simulink model "BZERO_MODEL"  (R2025b)
settings: Solver=ode23t  StartTime=0.0  StopTime=10000  RelTol=1e-3
InitFcn:
  | setup_bzero;
values from neighbouring files (symbols this model uses):
  bike_mass = 220    [setup_bzero.m]
  finish_line = track_dist(end)    [setup_bzero.m]
  g = 9.81    [Fly_lap.m]    (also in setup_bzero.m)
  L = 2    [setup_bzero.m]
  Max_brake_pressure_F_Bar = 70    [setup_bzero.m]
  Max_brake_pressure_R_Bar = 20    [setup_bzero.m]
  mot_rpm_vec = [0, 250, 500, 750, 1000, 1250, 1500, 1750, 2000, 2250, 2500, 2750, 3000, 3250, 3500, 3750, 4000, 4250, 4500, 4750, 5000, 5250, 5500, 5750, 6000, 6250, 6500, 6750, 7000, 7250, 7500]    [setup_bzero.m]
  mot_trq_vec = [120, 120, 120, 120, 120, 120, 120, 120, 120, 120, 120, 120, 120, 120, 120, 120, 114.592, 107.851, 101.859, 96.498, 91.673, 87.308, 83.339, 79.716, 76.394, 73.339, 70.518, 67.906, 65.481, 63.223, 61.115]    [setup_bzero.m]
  Np = 12    [setup_bzero.m]
  Ns = 28    [setup_bzero.m]
  regen_bias = 0.2    [setup_bzero.m]
  s = surf(X_surf, Y_surf, Z_surf, Z_surf)    [Fly_lap.m]
  target_vel = data.Velocity_ms    [setup_bzero.m]
  track_dist = data.Distance_m    [setup_bzero.m]
  track_grade = data.Grade_rad    [setup_bzero.m]
  V_init = 117    [setup_bzero.m]
  v_init = target_vel(1)    [setup_bzero.m]
undefined symbols (not defined in the file or in its folder): Driver_Ki, Driver_Kp, Neg, Pos
libraries: fl_lib x20, nesl_utility x13, sdl_lib x7, batteryecm_lib x1, autolibshared x1
(part 2 of 2)

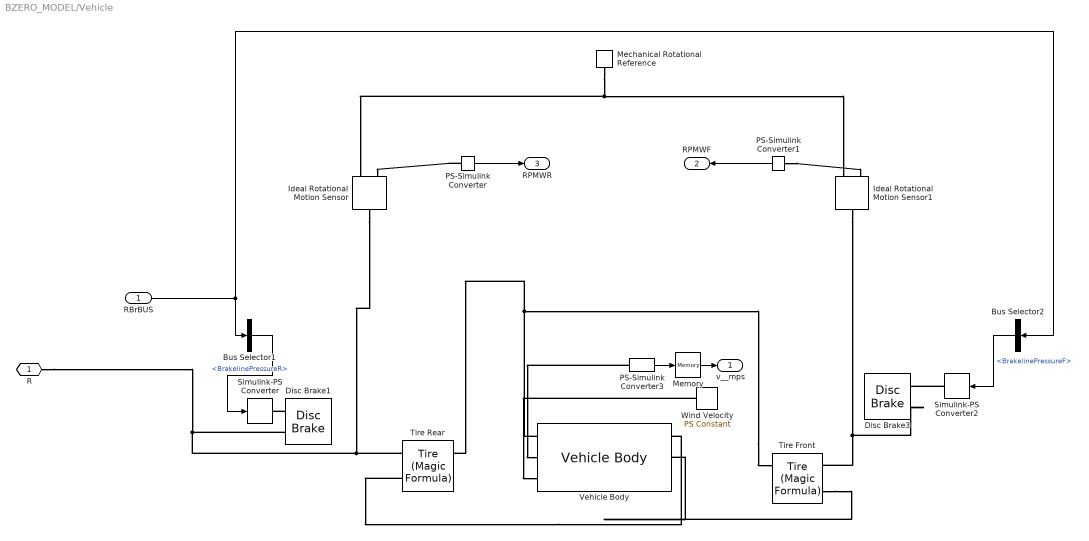
== system BZERO_MODEL/Vehicle ==
  RBrBUS : Inport
  Bus Selector1 : BusSelector  OutputSignals=BrakelinePressureR
  Bus Selector2 : BusSelector  OutputSignals=BrakelinePressureF
  Disc Brake1 : sdl_lib/Brakes & Detents/Rotational/Disc Brake  r_mean=R_eff m  bore=D_piston m  n_pads=2  thermal_port=simscape.enum.thermaleffects.omit  mu_static=Static_Cf  mu_coulomb=mu_pad  temperature_TLU=[280, 300, 320] K  mu_static_TLU=[.9, .8, .7]  mu_coulomb_TLU=[.8, .7, .6]  brkwy_vel=Break_Fric_v_rads rad/s  visc_coef=Viscous_Cf N*m*s/rad  thermal_mass=50 kJ/K  temperature_specify=off  temperature_priority=High  temperature=300 K  temperature_nominal_specify=off  temperature_nominal_value=1  temperature_nominal_unit=K
  Disc Brake3 : sdl_lib/Brakes & Detents/Rotational/Disc Brake  r_mean=R_eff m  bore=D_piston m  n_pads=2  thermal_port=simscape.enum.thermaleffects.omit  mu_static=Static_Cf  mu_coulomb=mu_pad  temperature_TLU=[280, 300, 320] K  mu_static_TLU=[.9, .8, .7]  mu_coulomb_TLU=[.8, .7, .6]  brkwy_vel=Break_Fric_v_rads rad/s  visc_coef=Viscous_Cf N*m*s/rad  thermal_mass=50 kJ/K  temperature_specify=off  temperature_priority=High  temperature=300 K  temperature_nominal_specify=off  temperature_nominal_value=1  temperature_nominal_unit=K
  Ideal Rotational Motion Sensor : fl_lib/Mechanical/Mechanical Sensors/Ideal Rotational Motion Sensor  reference=foundation.enum.MeasurementReference.difference  acceleration_port=false  velocity_port=true  position_port=false  wrap_angle=false  offset=0 rad
      settings: InternalSimscapePortConfiguration="{\"Bottom\":[],\"Left\":[{\"id\":\"R\",\"label\":\"R\",\"type\":\"foundation.mechanical.rotational.rotational\"}],\"Right\":[{\"id\":\"C\",\"label\":\"C\",\"type\":\"foundation.mechanical.rotational.rotational\"},{\"id\":\"W\",\"label\":\"W\",\"type\":\"output\"}],\"Top\":[]}"
  Ideal Rotational Motion Sensor1 : fl_lib/Mechanical/Mechanical Sensors/Ideal Rotational Motion Sensor  reference=foundation.enum.MeasurementReference.difference  acceleration_port=false  velocity_port=true  position_port=false  wrap_angle=false  offset=0 rad
      settings: InternalSimscapePortConfiguration="{\"Bottom\":[],\"Left\":[{\"id\":\"R\",\"label\":\"R\",\"type\":\"foundation.mechanical.rotational.rotational\"}],\"Right\":[{\"id\":\"C\",\"label\":\"C\",\"type\":\"foundation.mechanical.rotational.rotational\"},{\"id\":\"W\",\"label\":\"W\",\"type\":\"output\"}],\"Top\":[]}"
  Mechanical Rotational Reference : fl_lib/Mechanical/Rotational Elements/Mechanical Rotational Reference
  Memory : Memory  InitialCondition=v_init  LinearizeMemory=on  LinearizeAsDelay=on
  PS-Simulink Converter : nesl_utility/PS-Simulink Converter  PhysicalDomain=network_engine_domain  SubClassName=ps_output  LeftPortType=input  RightPortType=output  PseudoPeriodic=off  Frequencies=[]  VectorFormat=inherit  Unit=rpm  AffineConversion=off
  PS-Simulink Converter1 : nesl_utility/PS-Simulink Converter  PhysicalDomain=network_engine_domain  SubClassName=ps_output  LeftPortType=input  RightPortType=output  PseudoPeriodic=off  Frequencies=[]  VectorFormat=inherit  Unit=rpm  AffineConversion=off
  PS-Simulink Converter3 : nesl_utility/PS-Simulink Converter  PhysicalDomain=network_engine_domain  SubClassName=ps_output  LeftPortType=input  RightPortType=output  PseudoPeriodic=off  Frequencies=[]  VectorFormat=1-D array  Unit=m/s  AffineConversion=off
  Simulink-PS Converter : nesl_utility/Simulink-PS Converter  PhysicalDomain=network_engine_domain  SubClassName=ps_input  LeftPortType=input  RightPortType=output  PseudoPeriodic=off  Frequencies=[]  NoiseDistribution=none  NoiseParameters=[]  Unit=Pa  AffineConversion=off  FilteringAndDerivatives=zero  SimscapeFilterOrder=1  InputFilterTimeConstant=.001  UdotUserProvided=0
  Simulink-PS Converter2 : nesl_utility/Simulink-PS Converter  PhysicalDomain=network_engine_domain  SubClassName=ps_input  LeftPortType=input  RightPortType=output  PseudoPeriodic=off  Frequencies=[]  NoiseDistribution=none  NoiseParameters=[]  Unit=Pa  AffineConversion=off  FilteringAndDerivatives=zero  SimscapeFilterOrder=1  InputFilterTimeConstant=.001  UdotUserProvided=0
  Tire Front : sdl_lib/Tires & Vehicles/Tire (Magic Formula)  parameterization=sdl.enum.magic_tire_model.peak  F_z1=Fz_rated N  F_x1=Fx_peak N  kappa1=slip_peak  B_m=10  C_m=1.9  D_m=1  E_m=0.97  fz0=4e+3 N  p_Cx=1.685  p_Dx=[ 1.21 -0.037 ]  p_Ex=[ 0.344 0.095 -0.02 0 ]  p_Kx=[ 21.51 -0.163 0.245 ]  p_Hx=[ -0.002 0.002 ]  p_Vx=[ 0 0 ]  rolling_radius_model=sdl.enum.RollingRadiusParameterization.Constant  r_e=wheel_radius m  r_0=0.3 m  breff=8.39  dreff=0.26  freff=0.074  q_re0=0.99  q_v1=0.008  longvl=17 m/s  cz=5e5 N/m  model_resistance=true  resistance_model=1  coeff=Ad  p_tire=2.5e+5 Pa  alpha=-0.003  beta=0.97  coeff_a=0.008399999999999999  coeff_b=6.2e-4 s/m  coeff_c=1.6e-4 s^2/m^2  p_tire0=240e3 Pa  fz0_resistance=4000 N  vH0=16 m/s  q_Sy=[.0082, 0, .0014, .001, 0, 0, 1.08, -.5]  v_thr=0.001 m/s  enable_scaling_coefficients=false  lfzO=1  lcx=1  lmux=1  lex=1  lkx=1  lhx=1  lvx=1  lmy=1  model_compliance=sdl.enum.compliance.off  stiffness=1e+6 N/m  damping=1000 N/(m/s)  model_inertia=1  inertia=I_wheel_front kg*m^2  initial_velocity=wheel_rpm_init rpm  vxlow=0.1 m/s  v_tr_thr=0.1*(0.1) m/s  kpumin=-1e5  kpumax=1e8
  Tire Rear : sdl_lib/Tires & Vehicles/Tire (Magic Formula)  parameterization=sdl.enum.magic_tire_model.peak  F_z1=Fz_rated N  F_x1=Fx_peak N  kappa1=slip_peak  B_m=10  C_m=1.9  D_m=1  E_m=0.97  fz0=4e+3 N  p_Cx=1.685  p_Dx=[ 1.21 -0.037 ]  p_Ex=[ 0.344 0.095 -0.02 0 ]  p_Kx=[ 21.51 -0.163 0.245 ]  p_Hx=[ -0.002 0.002 ]  p_Vx=[ 0 0 ]  rolling_radius_model=sdl.enum.RollingRadiusParameterization.Constant  r_e=wheel_radius m  r_0=0.3 m  breff=8.39  dreff=0.26  freff=0.074  q_re0=0.99  q_v1=0.008  longvl=17 m/s  cz=5e5 N/m  model_resistance=true  resistance_model=sdl.enum.rollingResistanceParameterization.constant  coeff=Ad  p_tire=2.5e+5 Pa  alpha=-0.003  beta=0.97  coeff_a=0.008399999999999999  coeff_b=6.2e-4 s/m  coeff_c=1.6e-4 s^2/m^2  p_tire0=240e3 Pa  fz0_resistance=4000 N  vH0=16 m/s  q_Sy=[.0082, 0, .0014, .001, 0, 0, 1.08, -.5]  v_thr=0.001 m/s  enable_scaling_coefficients=false  lfzO=1  lcx=1  lmux=1  lex=1  lkx=1  lhx=1  lvx=1  lmy=1  model_compliance=sdl.enum.compliance.off  stiffness=1e+6 N/m  damping=1000 N/(m/s)  model_inertia=1  inertia=I_wheel_rear kg*m^2  initial_velocity=wheel_rpm_init rpm  vxlow=0.1 m/s  v_tr_thr=0.1*(0.1) m/s  kpumin=-1e5  kpumax=1e8
  Vehicle Body : sdl_lib/Tires & Vehicles/Vehicle Body  mass=bike_mass kg  n_w=1  x_f=D_CoG_F_m m  x_r=D_CoG_R_m m  y_c=H_CoG_m m  mass_var=simscape.enum.onoff.off  g=g m/s^2  liftoff_warning=0  area=frontal_area m^2  Cd_var=false  Cd=cd_coeff  rho=rho kg/m^3  model_pitch=false  inertia=4000 kg*m^2  suspension_model=1  k_f=1e4 N/m  b_f=1e4 N/(m/s)  k_r=1e4 N/m  b_r=1e4 N/(m/s)  k_f_TLU=[-2000, -1000, 0, 1000, 2000] N  x_f_TLU=[-.4, -.2, 0, .2, .4] m  b_f_TLU=[-200, -100, 0, 100, 200] N  v_f_TLU=[-4, -2, 0, 2, 4] m/s  k_r_TLU=[-2000, -1000, 0, 1000, 2000] N  x_r_TLU=[-.4, -.2, 0, .2, .4] m  b_r_TLU=[-200, -100, 0, 100, 200] N  v_r_TLU=[-4, -2, 0, 2, 4] m/s  interp_method=simscape.enum.interpolation.linear  extrap_method=simscape.enum.extrapolation.linear  model_hardstop=0  upper_bound_f=.25 m  lower_bound_f=-.25 m  stop_k_f=1e6 N/m  stop_b_f=150 N/(m/s)  upper_bound_r=.25 m  lower_bound_r=-.25 m  stop_k_r=1e6 N/m  stop_b_r=150 N/(m/s)  initial_pitch=0 rad  initial_pitch_rate=0 rad/s  v_specify=on  v_priority=High  v=v_init m/s  v_nominal_specify=off  v_nominal_value=1  v_nominal_unit=m/s
      settings: InternalSimscapePortConfiguration="{\"Bottom\":[{\"id\":\"NR\",\"label\":\"NR\",\"type\":\"output\"},{\"id\":\"NF\",\"label\":\"NF\",\"type\":\"output\"},{\"id\":\"beta\",\"label\":\"beta\",\"type\":\"input\"}],\"Left\":[{\"id\":\"H\",\"label\":\"H\",\"type\":\"foundation.mechanical.translational.translational\"}],\"Right\":[],\"Top\":[{\"id\":\"V\",\"label\":\"V\",\"type\":\"output\"},{\"id\":\"wind\",\"label\":\"W\",\"type\":\"input\"}]}"
  Wind Velocity : fl_lib/Physical Signals/Sources/PS Constant  constant=0
  R : PMIOPort  Side=Left
  v__mps : Outport  VectorParamsAs1DForOutWhenUnconnected=off
  RPMWF : Outport  Port=2
  RPMWR : Outport  Port=3
  wires:
  RBrBUS/1 -> Bus Selector1/1, Bus Selector2/1
  Bus Selector1/1 -> Simulink-PS Converter/1  "<BrakelinePressureR>"
  PS-Simulink Converter3/1 -> Memory/1
  Memory/1 -> v__mps/1
  Bus Selector2/1 -> Simulink-PS Converter2/1  "<BrakelinePressureF>"
  PS-Simulink Converter/1 -> RPMWR/1
  PS-Simulink Converter1/1 -> RPMWF/1
  connections:
  Tire Rear/LConn1 -- Vehicle Body/RConn1
  Disc Brake1/LConn2 -- Tire Rear/LConn2 -- Ideal Rotational Motion Sensor/LConn1 -- R/RConn1
  Tire Front/LConn1 -- Vehicle Body/RConn2
  PS-Simulink Converter3/LConn1 -- Vehicle Body/LConn2
  Wind Velocity/RConn1 -- Vehicle Body/LConn3
  Vehicle Body/LConn1 -- Tire Rear/RConn2 -- Tire Front/RConn2
  Disc Brake3/LConn2 -- Ideal Rotational Motion Sensor1/LConn1 -- Tire Front/LConn2
  Disc Brake1/LConn1 -- Simulink-PS Converter/RConn1
  Simulink-PS Converter2/RConn1 -- Disc Brake3/LConn1
  Mechanical Rotational Reference/LConn1 -- Ideal Rotational Motion Sensor/RConn1 -- Ideal Rotational Motion Sensor1/RConn1
  PS-Simulink Converter/LConn1 -- Ideal Rotational Motion Sensor/RConn2
  PS-Simulink Converter1/LConn1 -- Ideal Rotational Motion Sensor1/RConn2

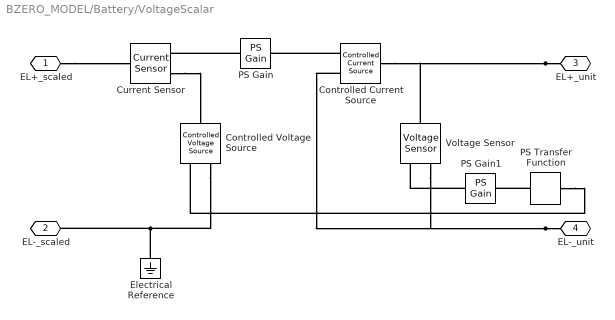
== system BZERO_MODEL/Battery/VoltageScalar ==
  Controlled Current Source : fl_lib/Electrical/Electrical Sources/Controlled Current Source
  Controlled Voltage Source : fl_lib/Electrical/Electrical Sources/Controlled Voltage Source
  Current Sensor : fl_lib/Electrical/Electrical Sensors/Current Sensor
  Electrical Reference : fl_lib/Electrical/Electrical Elements/Electrical Reference
  PS Gain : fl_lib/Physical Signals/Functions/PS Gain  gain=1/n_para
  PS Gain1 : fl_lib/Physical Signals/Functions/PS Gain  gain=n_ser
  PS Transfer Function : fl_lib/Physical Signals/Linear Operators/PS Transfer Function  transfer_function_type=foundation.enum.transfer_function_type.lag  T=t_filt s  T1=2 s  T2=1 s  reset_method=foundation.enum.IntegratorResetSpec.None  initial_condition_spec=foundation.enum.IntegratorICSpec.Internal  y0=V_init*n_ser V
      settings: InternalSimscapePortConfiguration="{\"Bottom\":[],\"Left\":[{\"id\":\"U\",\"label\":\"\",\"type\":\"input\"}],\"Right\":[{\"id\":\"Y\",\"label\":\"\",\"type\":\"output\"}],\"Top\":[]}"
  Voltage Sensor : fl_lib/Electrical/Electrical Sensors/Voltage Sensor
  EL+_scaled : PMIOPort  Side=Left
  EL-_scaled : PMIOPort  Port=2  Side=Left
  EL+_unit : PMIOPort  Port=3  Side=Right
  EL-_unit : PMIOPort  Port=4  Side=Right
  connections:
  EL+_scaled/RConn1 -- Current Sensor/LConn1
  Current Sensor/RConn2 -- Controlled Voltage Source/LConn1
  Controlled Voltage Source/RConn2 -- Electrical Reference/LConn1 -- EL-_scaled/RConn1
  PS Gain/LConn1 -- Current Sensor/RConn1
  Controlled Current Source/RConn1 -- PS Gain/RConn1
  EL+_unit/RConn1 -- Controlled Current Source/LConn1 -- Voltage Sensor/LConn1
  EL-_unit/RConn1 -- Controlled Current Source/RConn2 -- Voltage Sensor/RConn2
  PS Gain1/LConn1 -- Voltage Sensor/RConn1
  PS Transfer Function/LConn1 -- PS Gain1/RConn1
  PS Transfer Function/RConn1 -- Controlled Voltage Source/RConn1

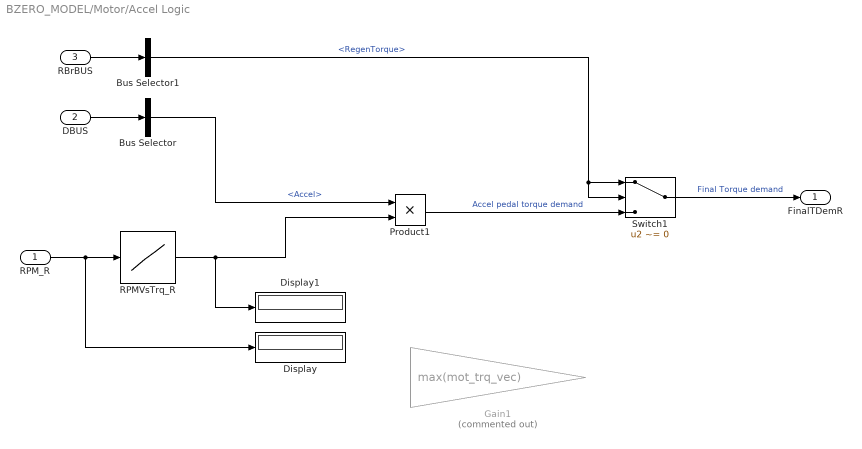
== system BZERO_MODEL/Motor/Accel Logic ==
  RPM_R : Inport
  DBUS : Inport  Port=2
  RBrBUS : Inport  Port=3
  Bus Selector : BusSelector  OutputSignals=Info.Accel
  Bus Selector1 : BusSelector  OutputSignals=RegenTorque
  Display : Display
  Display1 : Display
  Gain1 : Gain  Commented=on  Gain=max(mot_trq_vec)
  Product1 : Product
  RPMVsTrq_R : Lookup_n-D  NumberOfTableDimensions=1  BreakpointsForDimension1=mot_rpm_vec  Table=mot_trq_vec  ExtrapMethod=Clip  InternalRulePriority=Speed  RndMeth=Simplest
  Switch1 : Switch  Criteria=u2 ~= 0  SaturateOnIntegerOverflow=off  InputSameDT=off
  FinalTDemR : Outport
  wires:
  DBUS/1 -> Bus Selector/1
  Bus Selector/1 -> Product1/1  "<Accel>"
  RBrBUS/1 -> Bus Selector1/1
  Bus Selector1/1 -> Switch1/2, Switch1/1  "<RegenTorque>"
  Product1/1 -> Switch1/3  "Accel pedal torque demand"
  Switch1/1 -> FinalTDemR/1  "Final Torque demand"
  RPM_R/1 -> RPMVsTrq_R/1, Display/1
  RPMVsTrq_R/1 -> Display1/1, Product1/2

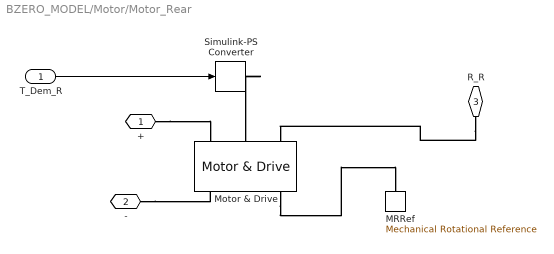
== system BZERO_MODEL/Motor/Motor_Rear ==
  T_Dem_R : Inport
  MRRef : fl_lib/Mechanical/Rotational Elements/Mechanical Rotational Reference
  Motor & Drive : sdl_lib/Engines & Motors/Motor & Drive  torque_max=max(mot_trq_vec) N*m  power_max=Max_power_motor_R_W W  Tc=Torque_control_T s  eff=Motor_eff_R  w_eff=RPM_measure_eff_R_RPM rpm  T_eff=Torque_measure_eff_R_Nm N*m  thermal_port=simscape.enum.thermaleffects.omit  thermal_mass=100 J/K  temperature_specify=off  temperature_priority=High  temperature=300 K  temperature_nominal_specify=off  temperature_nominal_value=1  temperature_nominal_unit=K
      settings: InternalSimscapePortConfiguration="{\"Bottom\":[],\"Left\":[{\"id\":\"Vp\",\"label\":\"+\",\"type\":\"foundation.electrical.electrical\"},{\"id\":\"Tr\",\"label\":\"Tr\",\"type\":\"input\"},{\"id\":\"R\",\"label\":\"R\",\"type\":\"foundation.mechanical.rotational.rotational\"}],\"Right\":[{\"id\":\"Vm\",\"label\":\"-\",\"type\":\"foundation.electrical.electrical\"},{\"id\":\"Omega\",\"label\":\"w\",\"type\":\"output\"},{\"id\":\"C\",\"label\":\"C\",\"type\":\"foundation.mechanical.rotational.rotational\"}],\"Top\":[]}"
  Simulink-PS Converter : nesl_utility/Simulink-PS Converter  PhysicalDomain=network_engine_domain  SubClassName=ps_input  LeftPortType=input  RightPortType=output  PseudoPeriodic=off  Frequencies=[]  NoiseDistribution=none  NoiseParameters=[]  Unit=N*m  AffineConversion=off  FilteringAndDerivatives=zero  SimscapeFilterOrder=1  InputFilterTimeConstant=.001  UdotUserProvided=0
  + : PMIOPort  Side=Left
  - : PMIOPort  Port=2  Side=Left
  R_R : PMIOPort  Port=3  Side=Right
  wires:
  T_Dem_R/1 -> Simulink-PS Converter/1
  connections:
  Motor & Drive/RConn3 -- MRRef/LConn1
  Simulink-PS Converter/RConn1 -- Motor & Drive/LConn2
  +/RConn1 -- Motor & Drive/LConn1
  -/RConn1 -- Motor & Drive/RConn1
  R_R/RConn1 -- Motor & Drive/LConn3
